simulink model "Delta_Inshallah_15RAMADAN_Circular"  (R2023b)
settings: Solver=VariableStepAuto  StartTime=0  StopTime=0.6  FixedStep=1  RelTol=1e-3
model workspace: external: MATLAB File D:\College\Senior 2\GP\Delta\Design\INSHALLAAHHHHH\SSCPE\25Mar\Ignorant_DataFile.m (data not in the file)
values from neighbouring files (symbols this model uses):
  X = [0 -180 -180 -180 180 180 180 180 0]    [Simulaiton_Main.m]    (also in csp_XYZ.m; csp_XYZ_X.m = [-180 -180]; csp_XYZ_circular_motion.m = center(1) + radius * cos(theta); csp_angles.m)
  Y = zeros(1,numel(X_3ars))    [CSPPPPPPPPPPPPpp.m]    (also in Simulaiton_Main.m = zeros(1,9); csp_XYZ.m = zeros(1,9); csp_XYZ_X.m = [0 0]; csp_XYZ_circular_motion.m = center(2) + radius * sin(theta))
  Z = -400*ones(1,numel(X_3ars))    [CSPPPPPPPPPPPPpp.m]    (also in Simulaiton_Main.m = [-300 -300 -400 -300 -300 -300 -400 -300 -300]; csp_XYZ.m = [-300 -300 -400 -300 -300 -300 -400 -300 -300]; csp_XYZ_X.m = [-300 -500]; csp_XYZ_circular_motion.m = center(3) * ones(size(X)))
undefined symbols (not defined in the file or in its folder): smiData
libraries: sm_lib x390, nesl_utility x4, simulink_extras x1
(part 1 of 8)
settings Model: Creator=Dell  LastModifiedBy=Dell
settings SolverCC: EnableFixedStepZeroCrossing=on

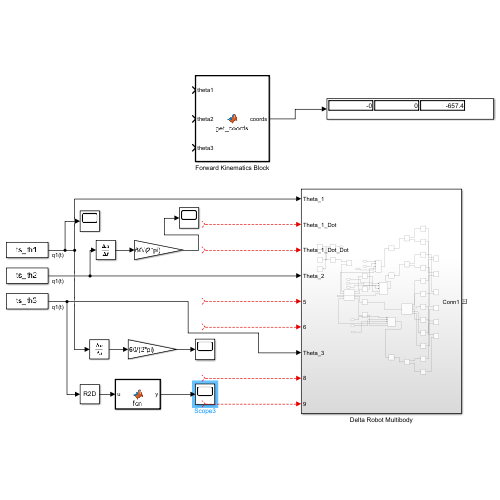
[thumbnail: Simulink's stored preview of the top-level diagram]
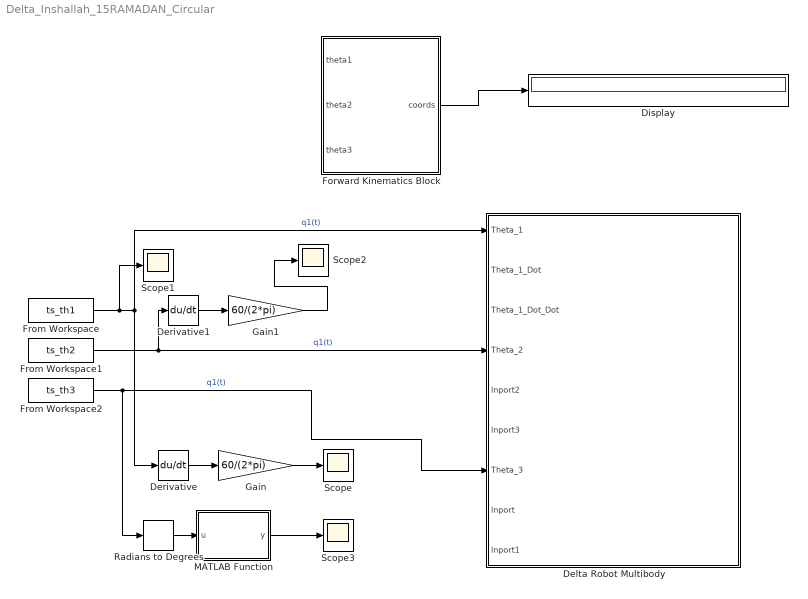
== system Delta_Inshallah_15RAMADAN_Circular ==
  Delta Robot Multibody : Subsystem
  Derivative : Derivative
  Derivative1 : Derivative
  Display : Display
  Forward Kinematics Block : MATLAB Function  TreatAsAtomicUnit=on
  From Workspace : FromWorkspace  VariableName=ts_th1
  From Workspace1 : FromWorkspace  VariableName=ts_th2
  From Workspace2 : FromWorkspace  VariableName=ts_th3
  Gain : Gain  Gain=60/(2*pi)
  Gain1 : Gain  Gain=60/(2*pi)
  MATLAB Function : MATLAB Function  TreatAsAtomicUnit=on
  Radians to Degrees : simulink_extras/Transformations/Radians to Degrees
  Scope{,1..3} (4 alike) : Scope
  wires:
  Forward Kinematics Block/1(coords) -> Display/1
  ? -> Delta Robot Multibody/2(Theta_1_Dot)
  ? -> Delta Robot Multibody/3(Theta_1_Dot_Dot)
  ? -> Delta Robot Multibody/5(Inport2)
  ? -> Delta Robot Multibody/6(Inport3)
  ? -> Delta Robot Multibody/8(Inport)
  ? -> Delta Robot Multibody/9(Inport1)
  From Workspace/1 -> Delta Robot Multibody/1(Theta_1), Derivative/1, Scope1/1  "q1(t)"
  From Workspace1/1 -> Derivative1/1, Delta Robot Multibody/4(Theta_2)  "q1(t)"
  From Workspace2/1 -> Radians to Degrees/1, Delta Robot Multibody/7(Theta_3)  "q1(t)"
  Gain/1 -> Scope/1
  Derivative/1 -> Gain/1
  Derivative1/1 -> Gain1/1
  Gain1/1 -> Scope2/1
  Radians to Degrees/1 -> MATLAB Function/1(u)
  MATLAB Function/1(y) -> Scope3/1
